simulink library "Libreria"  (R2019a)
settings: Solver=VariableStepAuto  StartTime=0.0  StopTime=10.0  RelTol=1e-3
values from neighbouring files (symbols this model uses):
  T_muestreo = 1    [Inicializacion_datos_distrito_personalizado.m]    (also in Inicializacion_datos_invernadero_tradicional.m; Inicializacion_datos_microred.m; Inicializacion_datos_nanofiltracion.m; Inicializacion_datos_oficinas.m)
undefined symbols (not defined in the file or in its folder): beta1, dispatch_factor, efficiency, Max_in, Min_in, Tm
settings Model: Creator=Usuario  LastModifiedBy=Jero

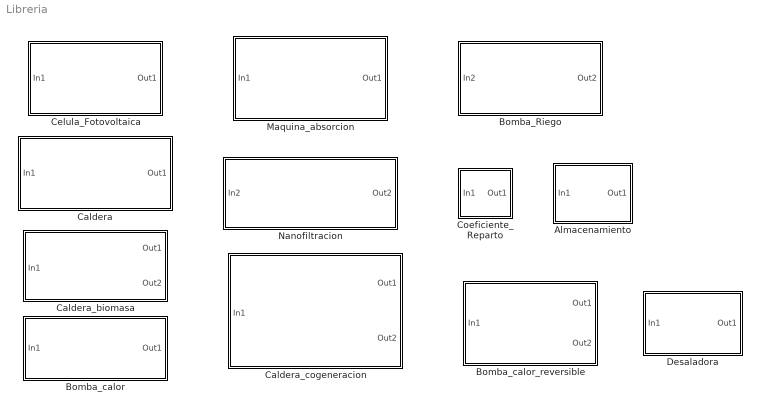
== system Libreria ==
  Almacenamiento : Subsystem  mask{Up2=1000, Low2=0, r_c=1, Up=1000, Low=0, r_d=1, Up1=1000, Low1=0, almacenamiento_inicial=0, cpa=1, almacenamiento_on=on}
      mask prompts: Up2 "Máximo"; Low2 "Mínimo"; r_c "rendimiento"; Up "Máximo"; Low "Mínimo"; r_d "rendimiento"; Up1 "Máximo"; Low1 "Mínimo"; almacenamiento_inicial "Condiciones iniciales"; cpa "Coeficiente de pérdidas"; almacenamiento_on "Almacenar energía"
      mask DialogControl DescGroupVar Prompt: Descripción
      mask DialogControl DescTextVar Prompt: Bloque de almacenamiento: se coloca en serie con la salida
      mask DialogControl ParameterGroupVar Prompt: Límites de los flujos de energía
      mask DialogControl Container6 Prompt: Carga
      mask DialogControl Container3 Prompt: Descarga
      mask DialogControl Container8 Prompt: Almacenamiento
      mask Display:
      | Ud = get_param(gcb,'UserData');
      | image(Ud.icono);
      | color('red');
  Bomba_Riego : Subsystem  mask{efficiency=1, dispatch_factor=beta1, T_muestreo=T_muestreo, Max_in=150, Max_out=150, n_salida=[0]}
      mask prompts: efficiency "Eficiencia"; dispatch_factor "Coeficiente de reparto"; T_muestreo "Tiempo de muestreo"; Max_in "Entrada"; Max_out "Salida"; n_salida "Salida asociada"
      mask TypeOptions efficiency: Ganancia_1_salida_max/efficiency
      mask TypeOptions dispatch_factor: Ganancia_1_salida_max/dispatch_factor
      mask TypeOptions T_muestreo: Ganancia_1_salida_max/T_muestreo
      mask TypeOptions Max_in: Ganancia_1_salida_max/Max_in
      mask DialogControl DescGroupVar Prompt: Descripción
      mask DialogControl DescTextVar Prompt: Su funcionamiento conlleva el uso de una demanda eléctrica en el energy hub. Representa el bombeamiento de agua para riego.
      mask DialogControl ParameterGroupVar Prompt: Parámetros
      mask DialogControl Container3 Prompt: Flujos máximos de energía
      mask DialogControl Container10 Prompt: Parámetros auxiliares
      mask Display:
      | ud=get_param(gcb,'UserData');
      | image(ud.icono);
      | color('green');
      | port_label('input',1,'IW');
      | port_label('output',1,'IW');
  Bomba_calor : Subsystem  mask{efficiency=[5.4], dispatch_factor=1, Tm=T_muestreo, Max_in=10, Max_out=54}
      mask prompts: efficiency "Eficiencia"; dispatch_factor "Coeficiente de reparto"; Tm "Tiempo de muestreo"; Max_in "Máximo"; Max_out "Máximo"
      mask TypeOptions efficiency: Ganancia_1_salida_max/efficiency
      mask TypeOptions dispatch_factor: Ganancia_1_salida_max/dispatch_factor
      mask TypeOptions Tm: Ganancia_1_salida_max/T_muestreo
      mask TypeOptions Max_in: Ganancia_1_salida_max/Max_in
      mask DialogControl DescGroupVar Prompt: Descripción
      mask DialogControl DescTextVar Prompt: Transforma energía eléctrica en calefacción.
      mask DialogControl ParameterGroupVar Prompt: Parámetros
      mask DialogControl Container3 Prompt: Límites de los flujos de energía
      mask DialogControl Container4 Prompt: Entrada
      mask DialogControl Container5 Prompt: Salida
      mask Display:
      | ud=get_param(gcb,'UserData');
      | image(ud.icono);
      | color('green');
      | port_label('input',1,'E');
      | color('red')
      | port_label('output',1,'H');
  Bomba_calor_reversible : Subsystem  mask{efficiency=efficiency, dispatch_factor=1, T_muestreo=T_muestreo, Max_in=Max_in, Min_in=Min_in, Max_out=[30 40], Salida_Binaria=[1 0]}
      mask prompts: efficiency "Eficiencia"; dispatch_factor "Coeficiente de reparto"; T_muestreo "Tiempo de muestreo"; Max_in "Máxima"; Min_in "Mínima"; Max_out "Máximo"; Salida_Binaria "Salidas Binarias:"
      mask TypeOptions efficiency: Ganancia_2_salidas/efficiency
      mask TypeOptions dispatch_factor: Ganancia_2_salidas/dispatch_factor
      mask TypeOptions T_muestreo: Ganancia_2_salidas/T_muestreo
      mask TypeOptions Max_in: Ganancia_2_salidas/Max_in
      mask TypeOptions Min_in: Ganancia_2_salidas/Min_in
      mask DialogControl DescGroupVar Prompt: Descripción
      mask DialogControl DescTextVar Prompt: Transforma energía eléctrica en refrigeración o calefacción. La transformación no se realiza simultáneamente.
      mask DialogControl ParameterGroupVar Prompt: Parámetros
      mask DialogControl Container3 Prompt: Límites de los flujos de energía
      mask DialogControl Container4 Prompt: Entrada
      mask DialogControl Container5 Prompt: Salida
      mask DialogControl Container6 Prompt: Parámetro auxiliar:
      mask DialogControl Control2 Prompt: Cambia durante la ejecución del optimizador. Sólo modifique este parámetro si va a realizar simulación sin optimizar previamente, en caso contrario no tendrá efecto la modificación.
      mask Display:
      | ud=get_param(gcb,'UserData');
      | image(ud.icono);
      | color('green');
      | port_label('input',1,'E');
      | color('blue');
      | port_label('output',1,'C');
      | color('red');
      | port_label('output',2,'H');
  Caldera : Subsystem  mask{efficiency=0, dispatch_factor=1, T_muestreo=T_muestreo, Min_in=0, Max_in=0, Max_out=1000}
      mask prompts: efficiency "Eficiencia"; dispatch_factor "Coeficiente de reparto"; T_muestreo "Tiempo de muestreo"; Min_in "Mínimo"; Max_in "Máximo"; Max_out "Máximo"
      mask TypeOptions efficiency: Ganancia_1_salida_max_min/efficiency
      mask TypeOptions dispatch_factor: Ganancia_1_salida_max_min/dispatch_factor
      mask TypeOptions T_muestreo: Ganancia_1_salida_max_min/T_muestreo
      mask TypeOptions Min_in: Ganancia_1_salida_max_min/Min_in
      mask TypeOptions Max_in: Ganancia_1_salida_max_min/Max_in
      mask DialogControl DescGroupVar Prompt: Descripción
      mask DialogControl DescTextVar Prompt: Transforma combustible en calefacción.
      mask DialogControl ParameterGroupVar Prompt: Parámetros
      mask DialogControl Container5 Prompt: Límites de los flujos de energía
      mask DialogControl Container6 Prompt: Entrada
      mask DialogControl Container7 Prompt: Salida
      mask Display:
      | Ud = get_param(gcb,'UserData');
      | image(Ud.icono);
      | color('black');
      | port_label('input',1,'F');
      | color('red')
      | port_label('output',1,'H');
  Caldera_biomasa : Subsystem  mask{efficiency=efficiency, dispatch_factor=dispatch_factor, T_muestreo=Tm, Max_in=Max_in, Min_in=Min_in, Max_out=0}
      mask prompts: efficiency "Eficiencia"; dispatch_factor "Coeficiente de reparto"; T_muestreo "Tiempo de muestreo"; Max_in "Entrada máxima"; Min_in "Entrada mínima"; Max_out "Máxima"
      mask TypeOptions efficiency: Ganancia_2_salidas/efficiency
      mask TypeOptions dispatch_factor: Ganancia_2_salidas/dispatch_factor
      mask TypeOptions T_muestreo: Ganancia_2_salidas/T_muestreo
      mask TypeOptions Max_in: Ganancia_2_salidas/Max_in
      mask TypeOptions Min_in: Ganancia_2_salidas/Min_in
      mask DialogControl DescGroupVar Prompt: Descripción
      mask DialogControl DescTextVar Prompt: Transforma el combustible en calefacción y captura el dióxido de carbono generado
      mask DialogControl ParameterGroupVar Prompt: Parámetros
      mask DialogControl Container7 Prompt: Flujos de energía
      mask DialogControl Container8 Prompt: Entrada
      mask DialogControl Container9 Prompt: Salida
      mask Display:
      | Ud = get_param(gcb,'UserData');
      | image(Ud.icono);
      | color('black');
      | port_label('input',1,'F');
      | color('red');
      | port_label('output',1,'H');
      | color('cyan');
      | port_label('output',2,'CO2');
  Caldera_cogeneracion : Subsystem  mask{efficiency=[10 10], dispatch_factor=1, Tm=T_muestreo, Max_in=1, Min_in=0, Max_out=[10 10]}
      mask prompts: efficiency "Eficiencia"; dispatch_factor "Coeficiente de reparto"; Tm "Tiempo de muestreo"; Max_in "Máxima"; Min_in "Mínima"; Max_out "Máxima"
      mask TypeOptions efficiency: Ganancia_2_salidas/efficiency
      mask TypeOptions dispatch_factor: Ganancia_2_salidas/dispatch_factor
      mask TypeOptions Tm: Ganancia_2_salidas/T_muestreo
      mask TypeOptions Max_in: Ganancia_2_salidas/Max_in
      mask TypeOptions Min_in: Ganancia_2_salidas/Min_in
      mask DialogControl DescGroupVar Prompt: Descripción
      mask DialogControl DescTextVar Prompt: Transforma combustible en energía eléctrica y calefacción simultáneamente.
      mask DialogControl ParameterGroupVar Prompt: Parámetros
      mask DialogControl Container3 Prompt: Flujos de energía
      mask DialogControl Container4 Prompt: Entrada
      mask DialogControl Container5 Prompt: Salida
      mask Display:
      | Ud = get_param(gcb,'UserData');
      | image(Ud.icono);
      | color('black');
      | port_label('input',1,'F');
      | color('green');
      | port_label('output',1,'E');
      | color('red');
      | port_label('output',2,'H');
  Celula_Fotovoltaica : Subsystem  mask{efficiency=[0.211], dispatch_factor=1, T_muestreo=T_muestreo, Max_in=1200, Max_out=2000}
      mask prompts: efficiency "Eficiencia"; dispatch_factor "Coeficiente de reparto"; T_muestreo "Tiempo de muestreo"; Max_in "Entrada"; Max_out "Salida"
      mask TypeOptions efficiency: Ganancia_1_salida_max/efficiency
      mask TypeOptions dispatch_factor: Ganancia_1_salida_max/dispatch_factor
      mask TypeOptions T_muestreo: Ganancia_1_salida_max/T_muestreo
      mask TypeOptions Max_in: Ganancia_1_salida_max/Max_in
      mask DialogControl DescGroupVar Prompt: Descripción
      mask DialogControl DescTextVar Prompt: En eficiencia se introduce el parámetro de eficiencia de cada panel y los flujos máximos son relativos a un panel.
      mask DialogControl ParameterGroupVar Prompt: Parámetros
      mask DialogControl Container3 Prompt: Flujos máximos
      mask Display:
      | Ud = get_param(gcb,'UserData');
      | image(Ud.icono);
      | color('yellow');
      | port_label('input',1,'R');
      | color('green');
      | port_label('output',1,'E');
  Coeficiente_Reparto : Subsystem  mask{dispatch_factor=1, Tm=T_muestreo, Max_out=inf, Max_in=inf, efficiency=1}
      mask prompts: dispatch_factor "Coeficiente de reparto"; Tm "Tiempo de muestreo"
      mask TypeOptions dispatch_factor: Funcion_coef_reparto/dispatch_factor
      mask TypeOptions Tm: Funcion_coef_reparto/Tm
      mask DialogControl DescGroupVar Prompt: Descripción
      mask DialogControl DescTextVar Prompt: Bloque Coeficiente de Reparto. Admite alfa o beta seguidos de un número: alfa1, alfa2...
      mask DialogControl ParameterGroupVar Prompt: Parámetros
      mask Display: disp('CR')
  Desaladora : Subsystem  mask{efficiency=1, dispatch_factor=beta1, T_muestreo=T_muestreo, Max_in=150, Max_out=150, n_salida=[0]}
      mask prompts: efficiency "Eficiencia"; dispatch_factor "Coeficiente de reparto"; T_muestreo "Tiempo de muestreo"; Max_in "Entrada"; Max_out "Salida"; n_salida "Salida asociada"
      mask TypeOptions efficiency: Ganancia_1_salida_max/efficiency
      mask TypeOptions dispatch_factor: Ganancia_1_salida_max/dispatch_factor
      mask TypeOptions T_muestreo: Ganancia_1_salida_max/T_muestreo
      mask TypeOptions Max_in: Ganancia_1_salida_max/Max_in
      mask DialogControl DescGroupVar Prompt: Descripción
      mask DialogControl DescTextVar Prompt: Su funcionamiento conlleva el uso de una demanda eléctrica en el energy hub. Representa el bombeamiento de agua para riego.
      mask DialogControl ParameterGroupVar Prompt: Parámetros
      mask DialogControl Container3 Prompt: Flujos máximos de energía
      mask DialogControl Container10 Prompt: Parámetros auxiliares
      mask Display:
      | ud=get_param(gcb,'UserData');
      | image(ud.icono);
      | color('green');
      | port_label('input',1,'SW');
      | color('cyan');
      | port_label('output',1,'IW');
  Maquina_absorcion : Subsystem  mask{efficiency=efficiency, dispatch_factor=1, Tm=T_muestreo, Min_in=Min_in, Max_in=Max_in, Max_out=70}
      mask prompts: efficiency "Eficiencia"; dispatch_factor "Coeficiente de reparto"; Tm "Tiempo de muestreo"; Min_in "Mínimo"; Max_in "Máximo"; Max_out "Máximo"
      mask TypeOptions efficiency: Ganancia_1_salida_max_min/efficiency
      mask TypeOptions dispatch_factor: Ganancia_1_salida_max_min/dispatch_factor
      mask TypeOptions Tm: Ganancia_1_salida_max_min/T_muestreo
      mask TypeOptions Min_in: Ganancia_1_salida_max_min/Min_in
      mask TypeOptions Max_in: Ganancia_1_salida_max_min/Max_in
      mask DialogControl DescGroupVar Prompt: Descripción
      mask DialogControl DescTextVar Prompt: Transforma calefacción en refrigeración mediante absorción
      mask DialogControl ParameterGroupVar Prompt: Parámetros
      mask DialogControl Container3 Prompt: Límites de los flujos de energía
      mask DialogControl Container4 Prompt: Entrada
      mask DialogControl Container5 Prompt: Salida
      mask Display:
      | ud=get_param(gcb,'UserData');
      | image(ud.icono);
      | color('blue');
      | port_label('output',1,'C');
      | color('red');
      | port_label('input',1,'H');
  Nanofiltracion : Subsystem  mask{efficiency=efficiency, dispatch_factor=beta1, T_muestreo=T_muestreo, Max_in=Max_in, Max_out=60, n_salida=0}
      mask prompts: efficiency "Eficiencia"; dispatch_factor "Coeficiente de reparto"; T_muestreo "Tiempo de muestreo"; Max_in "Entrada"; Max_out "Salida"; n_salida "Salida asociada"
      mask TypeOptions efficiency: Ganancia_1_salida_max/efficiency
      mask TypeOptions dispatch_factor: Ganancia_1_salida_max/dispatch_factor
      mask TypeOptions T_muestreo: Ganancia_1_salida_max/T_muestreo
      mask TypeOptions Max_in: Ganancia_1_salida_max/Max_in
      mask DialogControl DescGroupVar Prompt: Descripción
      mask DialogControl DescTextVar Prompt: Módulo de nanofiltración. Purifica el agua residual, potabilizándola. Debe de tener una salida asociada
      mask DialogControl ParameterGroupVar Prompt: Parámetros
      mask DialogControl Container3 Prompt: Flujos máximos de energía
      mask DialogControl Container4 Prompt: Parámetros auxiliares
      mask Display:
      | Ud = get_param(gcb,'UserData');
      | image(Ud.icono);
      | color('red');
      | port_label('input',1,'WW');
      | color('green')
      | port_label('output',1,'IW');

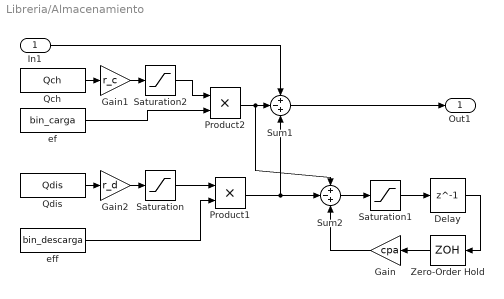
== system Libreria/Almacenamiento ==
  In1 : Inport
  Delay : Delay  DelayLength=1  InitialCondition=0
  Gain : Gain  Gain=cpa
  Gain1 : Gain  Gain=r_c
  Gain2 : Gain  Gain=r_d
  Product1 : Product
  Product2 : Product
  Qch : FromWorkspace  VariableName=Qch
  Qdis : FromWorkspace  VariableName=Qdis
  Saturation : Saturate  UpperLimit=Up  LowerLimit=Low
  Saturation1 : Saturate  UpperLimit=Up1  LowerLimit=Low1
  Saturation2 : Saturate  UpperLimit=Up2  LowerLimit=Low2
  Sum1 : Sum  Inputs=+-+
  Sum2 : Sum  Inputs=+-+
  Zero-Order Hold : ZeroOrderHold  SampleTime=-1
  ef : FromWorkspace  VariableName=bin_carga
  eff : FromWorkspace  VariableName=bin_descarga
  Out1 : Outport
  wires:
  Qdis/1 -> Gain2/1
  ef/1 -> Product2/2
  eff/1 -> Product1/2
  Saturation1/1 -> Delay/1
  In1/1 -> Sum1/1
  Sum1/1 -> Out1/1
  Sum2/1 -> Saturation1/1
  Delay/1 -> Zero-Order Hold/1
  Zero-Order Hold/1 -> Gain/1
  Gain/1 -> Sum2/3
  Qch/1 -> Gain1/1
  Gain1/1 -> Saturation2/1
  Gain2/1 -> Saturation/1
  Saturation/1 -> Product1/1
  Product1/1 -> Sum2/2, Sum1/3
  Saturation2/1 -> Product2/1
  Product2/1 -> Sum2/1, Sum1/2

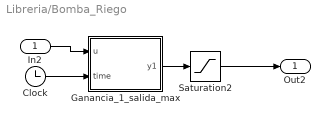
== system Libreria/Bomba_Riego ==
  In2 : Inport
  Clock : Clock
  Ganancia_1_salida_max : MATLAB Function  TreatAsAtomicUnit=on  mask{Max_in=Max_in, efficiency=efficiency, T_muestreo=T_muestreo, dispatch_factor=dispatch_factor}
      mask prompts: Max_in "Máximo"; efficiency "Eficiencia"; T_muestreo "Tiempo de muestreo"; dispatch_factor "Coeficiente de reparto"
  Saturation2 : Saturate  UpperLimit=Max_out  LowerLimit=-inf
  Out2 : Outport
  wires:
  Clock/1 -> Ganancia_1_salida_max/2(time)
  Saturation2/1 -> Out2/1
  In2/1 -> Ganancia_1_salida_max/1(u)
  Ganancia_1_salida_max/1(y1) -> Saturation2/1

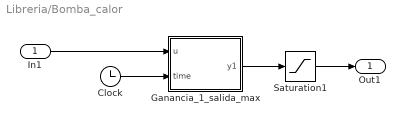
== system Libreria/Bomba_calor ==
  In1 : Inport
  Clock : Clock
  Ganancia_1_salida_max : MATLAB Function  TreatAsAtomicUnit=on  mask{Max_in=Max_in, efficiency=efficiency, T_muestreo=Tm, dispatch_factor=dispatch_factor}
      mask prompts: Max_in "Máximo"; efficiency "Eficiencia"; T_muestreo "Tiempo de muestreo"; dispatch_factor "Coeficiente de reparto"
  Saturation1 : Saturate  UpperLimit=Max_out(1)  LowerLimit=-inf
  Out1 : Outport
  wires:
  Saturation1/1 -> Out1/1
  Clock/1 -> Ganancia_1_salida_max/2(time)
  In1/1 -> Ganancia_1_salida_max/1(u)
  Ganancia_1_salida_max/1(y1) -> Saturation1/1

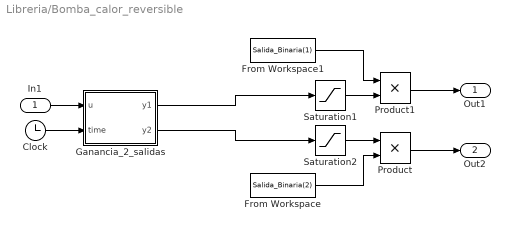
== system Libreria/Bomba_calor_reversible ==
  In1 : Inport
  Clock : Clock
  From Workspace : FromWorkspace  VariableName=Salida_Binaria(2)  SampleTime=0
  From Workspace1 : FromWorkspace  VariableName=Salida_Binaria(1)  SampleTime=0
  Ganancia_2_salidas : MATLAB Function  TreatAsAtomicUnit=on  mask{efficiency=efficiency, T_muestreo=T_muestreo, Max_in=Max_in, Min_in=Min_in, dispatch_factor=dispatch_factor}
      mask prompts: efficiency "Eficiencia"; T_muestreo "Tiempo de muestreo"; Max_in "Entrada máxima"; Min_in "Entrada mínima"; dispatch_factor "Coeficiente de reparto"
  Product : Product
  Product1 : Product
  Saturation1 : Saturate  UpperLimit=Max_out(1)  LowerLimit=-inf
  Saturation2 : Saturate  UpperLimit=Max_out(2)  LowerLimit=-inf
  Out1 : Outport
  Out2 : Outport  Port=2
  wires:
  In1/1 -> Ganancia_2_salidas/1(u)
  Clock/1 -> Ganancia_2_salidas/2(time)
  Ganancia_2_salidas/1(y1) -> Saturation1/1
  Ganancia_2_salidas/2(y2) -> Saturation2/1
  Product/1 -> Out2/1
  Saturation2/1 -> Product/1
  Saturation1/1 -> Product1/2
  Product1/1 -> Out1/1
  From Workspace/1 -> Product/2
  From Workspace1/1 -> Product1/1

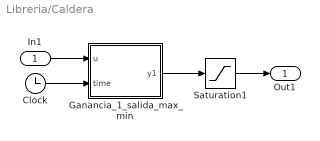
== system Libreria/Caldera ==
  In1 : Inport
  Clock : Clock
  Ganancia_1_salida_max_min : MATLAB Function  TreatAsAtomicUnit=on  mask{efficiency=efficiency, dispatch_factor=dispatch_factor, T_muestreo=T_muestreo, Min_in=Min_in, Max_in=Max_in}
      mask prompts: efficiency "Eficiencia"; dispatch_factor "Coeficiente de reparto"; T_muestreo "Tiempo de muestreo"; Min_in "Minimo de entrada"; Max_in "Minimo de salida"
  Saturation1 : Saturate  UpperLimit=Max_out  LowerLimit=-inf
  Out1 : Outport
  wires:
  Saturation1/1 -> Out1/1
  Ganancia_1_salida_max_min/1(y1) -> Saturation1/1
  Clock/1 -> Ganancia_1_salida_max_min/2(time)
  In1/1 -> Ganancia_1_salida_max_min/1(u)

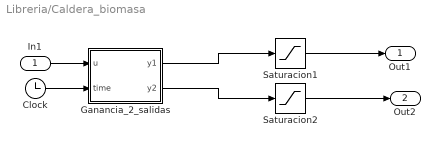
== system Libreria/Caldera_biomasa ==
  In1 : Inport
  Clock : Clock
  Ganancia_2_salidas : MATLAB Function  TreatAsAtomicUnit=on  mask{efficiency=efficiency, T_muestreo=T_muestreo, Max_in=Max_in, Min_in=Min_in, dispatch_factor=dispatch_factor}
      mask prompts: efficiency "Eficiencia"; T_muestreo "Tiempo de muestreo"; Max_in "Entrada máxima"; Min_in "Entrada mínima"; dispatch_factor "Coeficiente de reparto"
  Saturacion1 : Saturate  UpperLimit=Max_out(1)  LowerLimit=-inf
  Saturacion2 : Saturate  UpperLimit=Max_out(2)  LowerLimit=-inf
  Out1 : Outport
  Out2 : Outport  Port=2
  wires:
  Ganancia_2_salidas/2(y2) -> Saturacion2/1
  Ganancia_2_salidas/1(y1) -> Saturacion1/1
  Clock/1 -> Ganancia_2_salidas/2(time)
  In1/1 -> Ganancia_2_salidas/1(u)
  Saturacion2/1 -> Out2/1
  Saturacion1/1 -> Out1/1

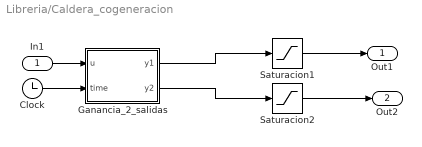
== system Libreria/Caldera_cogeneracion ==
  In1 : Inport
  Clock : Clock
  Ganancia_2_salidas : MATLAB Function  TreatAsAtomicUnit=on  mask{efficiency=efficiency, T_muestreo=Tm, Max_in=Max_in, Min_in=Min_in, dispatch_factor=dispatch_factor}
      mask prompts: efficiency "Eficiencia"; T_muestreo "Tiempo de muestreo"; Max_in "Entrada máxima"; Min_in "Entrada mínima"; dispatch_factor "Coeficiente de reparto"
  Saturacion1 : Saturate  UpperLimit=Max_out(1)  LowerLimit=-inf
  Saturacion2 : Saturate  UpperLimit=Max_out(2)  LowerLimit=-inf
  Out1 : Outport
  Out2 : Outport  Port=2
  wires:
  Saturacion1/1 -> Out1/1
  Saturacion2/1 -> Out2/1
  In1/1 -> Ganancia_2_salidas/1(u)
  Clock/1 -> Ganancia_2_salidas/2(time)
  Ganancia_2_salidas/1(y1) -> Saturacion1/1
  Ganancia_2_salidas/2(y2) -> Saturacion2/1

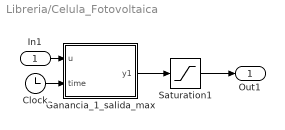
== system Libreria/Celula_Fotovoltaica ==
  In1 : Inport
  Clock : Clock
  Ganancia_1_salida_max : MATLAB Function  TreatAsAtomicUnit=on  mask{Max_in=Max_in, efficiency=efficiency, T_muestreo=T_muestreo, dispatch_factor=dispatch_factor}
      mask prompts: Max_in "Máximo"; efficiency "Eficiencia"; T_muestreo "Tiempo de muestreo"; dispatch_factor "Coeficiente de reparto"
  Saturation1 : Saturate  UpperLimit=Max_out  LowerLimit=-inf
  Out1 : Outport
  wires:
  Saturation1/1 -> Out1/1
  Ganancia_1_salida_max/1(y1) -> Saturation1/1
  In1/1 -> Ganancia_1_salida_max/1(u)
  Clock/1 -> Ganancia_1_salida_max/2(time)

== system Libreria/Coeficiente_Reparto ==
  In1 : Inport
  Clock : Clock
  Funcion_coef_reparto : MATLAB Function  TreatAsAtomicUnit=on  mask{dispatch_factor=dispatch_factor, Tm=Tm}
      mask prompts: dispatch_factor "Coeficiente de reparto"; Tm "Tiempo de muestreo"
  Out1 : Outport
  wires:
  In1/1 -> Funcion_coef_reparto/1(u)
  Clock/1 -> Funcion_coef_reparto/2(time)
  Funcion_coef_reparto/1(y) -> Out1/1

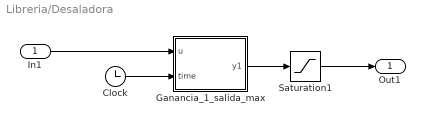
== system Libreria/Desaladora ==
  In1 : Inport
  Clock : Clock
  Ganancia_1_salida_max : MATLAB Function  TreatAsAtomicUnit=on  mask{Max_in=Max_in, efficiency=efficiency, T_muestreo=T_muestreo, dispatch_factor=dispatch_factor}
      mask prompts: Max_in "Máximo"; efficiency "Eficiencia"; T_muestreo "Tiempo de muestreo"; dispatch_factor "Coeficiente de reparto"
  Saturation1 : Saturate  UpperLimit=Max_out(1)  LowerLimit=-inf
  Out1 : Outport
  wires:
  In1/1 -> Ganancia_1_salida_max/1(u)
  Clock/1 -> Ganancia_1_salida_max/2(time)
  Ganancia_1_salida_max/1(y1) -> Saturation1/1
  Saturation1/1 -> Out1/1

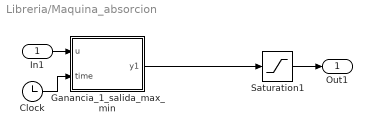
== system Libreria/Maquina_absorcion ==
  In1 : Inport
  Clock : Clock
  Ganancia_1_salida_max_min : MATLAB Function  TreatAsAtomicUnit=on  mask{efficiency=efficiency, dispatch_factor=dispatch_factor, T_muestreo=Tm, Min_in=Min_in, Max_in=Max_in}
      mask prompts: efficiency "Eficiencia"; dispatch_factor "Coeficiente de reparto"; T_muestreo "Tiempo de muestreo"; Min_in "Minimo de entrada"; Max_in "Minimo de salida"
  Saturation1 : Saturate  UpperLimit=Max_out  LowerLimit=-inf
  Out1 : Outport
  wires:
  In1/1 -> Ganancia_1_salida_max_min/1(u)
  Clock/1 -> Ganancia_1_salida_max_min/2(time)
  Ganancia_1_salida_max_min/1(y1) -> Saturation1/1
  Saturation1/1 -> Out1/1

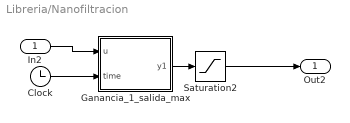
== system Libreria/Nanofiltracion ==
  In2 : Inport
  Clock : Clock
  Ganancia_1_salida_max : MATLAB Function  TreatAsAtomicUnit=on  mask{Max_in=Max_in, efficiency=efficiency, T_muestreo=T_muestreo, dispatch_factor=dispatch_factor}
      mask prompts: Max_in "Máximo"; efficiency "Eficiencia"; T_muestreo "Tiempo de muestreo"; dispatch_factor "Coeficiente de reparto"
  Saturation2 : Saturate  UpperLimit=Max_out  LowerLimit=-inf
  Out2 : Outport
  wires:
  Ganancia_1_salida_max/1(y1) -> Saturation2/1
  Saturation2/1 -> Out2/1
  In2/1 -> Ganancia_1_salida_max/1(u)
  Clock/1 -> Ganancia_1_salida_max/2(time)

== matlab function Libreria/Caldera/Ganancia_1_salida_max_min ==
  data: u input; y1 output; time input; Min_in parameter; Max_in parameter; efficiency parameter; T_muestreo parameter; dispatch_factor parameter
function y1  = fcn(u,time, Min_in, Max_in, efficiency, T_muestreo, dispatch_factor)
%efficiency: eficiencia
%Max_in: límite de entrada superior
%Min_in: límite de entrada inferior
%T_muestreo: tiempo de muestreo
%dispatch_factor: coeficiente de reparto
%time: tiempo de simulación
%u: entrada
%y1:salida
g=efficiency;
if(size(dispatch_factor,2)>1||size(g,1)>1)
    aux=floor(time/T_muestreo)+1;
    if(size(g,1)==1)
        u=min_max(u,dispatch_factor(aux),Max_in,Min_in)
        y1=u*dispatch_factor(aux)*g;
    end
    if(size(dispatch_factor,2)==1)
        u=min_max(u,dispatch_factor,Max_in,Min_in)
        y1=u*dispatch_factor*g(aux);
    end
else
    u=min_max(u,dispatch_factor,Max_in,Min_in)
    y1=u*dispatch_factor*g;
end
end

%obtengo los límites de entrada al dispositivo
function u=min_max(a,dispatch_factor,Max_in,Min_in)
if(a*dispatch_factor>Max_in)
    u=Max_in;
else
    u=a;
end
if(a*dispatch_factor<Min_in)
    u=Min_in;
else
    u=a;
end
end

== matlab function Libreria/Caldera_cogeneracion/Ganancia_2_salidas ==
  data: u input; y1 output; time input; y2 output; Min_in parameter; Max_in parameter; efficiency parameter; T_muestreo parameter; dispatch_factor parameter
function [y1,y2] = fcn(u,time, Min_in, Max_in, efficiency, T_muestreo, dispatch_factor)

%efficiency: eficiencia
%Max_in: límite de entrada superior
%Min_in: límite de entrada inferior
%T_muestreo: tiempo de muestreo
%dispatch_factor: coeficiente de reparto
%time: tiempo de simulación
%u: entrada
%y1: salida 1
%y2: salida 2

g=efficiency;
if(size(dispatch_factor,2)>1||size(g,1)>1)
    aux=floor(time/T_muestreo)+1;
    if(size(g,1)==1)
        u = max_min_u(u,dispatch_factor(aux),Min_in, Max_in);
        y1=u*dispatch_factor(aux)*g(1,1);
        y2=u*dispatch_factor(aux)*g(1,2);
    end
    if(size(dispatch_factor,2)==1)
        u = max_min_u(u,dispatch_factor, Min_in, Max_in);
        y1=u*dispatch_factor*g(aux,1);
        y2=u*dispatch_factor*g(aux,2);
    end
else
    u = max_min_u(u,dispatch_factor ,Min_in, Max_in);
    y1=u*dispatch_factor*g(1,1);
    y2=u*dispatch_factor*g(1,2);
end

end

% obtengo los límites de entrada de energía del dispositivo
function u = max_min_u(a,dispatch_factor, Min_in, Max_in)
if(a*dispatch_factor>Max_in)
    u=Max_in;
else
    u=a;
end
if(a*dispatch_factor<Min_in)
    u=Min_in;
else
    u=a;
end
end

== matlab function Libreria/Bomba_calor/Ganancia_1_salida_max ==
  data: u input; y1 output; time input; dispatch_factor parameter; T_muestreo parameter; efficiency parameter; Max_in parameter
function y1  = fcn(u,time, dispatch_factor, T_muestreo, efficiency, Max_in)
g=efficiency;

if(size(dispatch_factor,2)>1||size(g,1)>1)
    aux=floor(time/T_muestreo)+1;
    if(size(g,1)==1)
        u = max_min_u(u,dispatch_factor(aux), Max_in);
        y1=u*dispatch_factor(aux)*g;
    end
    if(size(dispatch_factor,2)==1)
        u = max_min_u(u,dispatch_factor,Max_in);
        y1=u*dispatch_factor*g(aux);
    end
else
    u = max_min_u(u,dispatch_factor,Max_in);
    y1=u*dispatch_factor*g;
end
end

% obtengo los límites de entrada de energía del dispositivo
function u = max_min_u(a,dispatch_factor,Max_in)
if(a*dispatch_factor>Max_in)
    u=Max_in;
else
    u=a;
end
end

== matlab function Libreria/Coeficiente_Reparto/Funcion_coef_reparto ==
  data: u input; y output; time input; dispatch_factor parameter; Tm parameter
function y = fcn(u,time, dispatch_factor, Tm)
%y: salida del bloque
%u: entrada 1 del bloque
%time: entrada 2 del bloque, tiempo de simulación
%dispatch_factor: vector coeficiente de reparto
%Tm: tiempo de muestreo
%Si el coeficiente de reparto no es un número
if(size(dispatch_factor,2)>1)
        %se obtiene la posición del vector en función del instante de muestreo
    aux=floor(time/Tm)+1;
    y=u*dispatch_factor(aux);
else
    %no se usa tiempo de muestreo
    y=u*dispatch_factor;
end

end

== matlab function Libreria/Maquina_absorcion/Ganancia_1_salida_max_min ==
  data: u input; y1 output; time input; Min_in parameter; Max_in parameter; efficiency parameter; T_muestreo parameter; dispatch_factor parameter
function y1  = fcn(u,time, Min_in, Max_in, efficiency, T_muestreo, dispatch_factor)
g=efficiency;
if(size(dispatch_factor,2)>1||size(g,1)>1)
    aux=floor(time/T_muestreo)+1;
    if(size(g,1)==1)
        u=min_max(u,dispatch_factor(aux),Max_in,Min_in)
        y1=u*dispatch_factor(aux)*g;
    end
    if(size(dispatch_factor,2)==1)
        u=min_max(u,dispatch_factor,Max_in,Min_in)
        y1=u*dispatch_factor*g(aux);
    end
else
    u=min_max(u,dispatch_factor,Max_in,Min_in)
    y1=u*dispatch_factor*g;
end
end

%obtengo los límites de entrada al dispositivo
function u=min_max(a,dispatch_factor,Max_in,Min_in)
if(a*dispatch_factor>Max_in)
    u=Max_in;
else
    u=a;
end
if(a*dispatch_factor<Min_in)
    u=Min_in;
else
    u=a;
end
end

== matlab function Libreria/Bomba_calor_reversible/Ganancia_2_salidas ==
  data: u input; y1 output; time input; y2 output; Min_in parameter; Max_in parameter; efficiency parameter; T_muestreo parameter; dispatch_factor parameter
function [y1,y2] = fcn(u,time, Min_in, Max_in, efficiency, T_muestreo, dispatch_factor)
g=efficiency;
if(size(dispatch_factor,2)>1||size(g,1)>1)
    aux=floor(time/T_muestreo)+1;
    if(size(g,1)==1)
        u = max_min_u(u,dispatch_factor(aux),Min_in, Max_in);
        y1=u*dispatch_factor(aux)*g(1,1);
        y2=u*dispatch_factor(aux)*g(1,2);
    end
    if(size(dispatch_factor,2)==1)
        u = max_min_u(u,dispatch_factor, Min_in, Max_in);
        y1=u*dispatch_factor*g(aux,1);
        y2=u*dispatch_factor*g(aux,2);
    end
else
    u = max_min_u(u,dispatch_factor ,Min_in, Max_in);
    y1=u*dispatch_factor*g(1,1);
    y2=u*dispatch_factor*g(1,2);
end

end

% obtengo los límites de entrada de energía del dispositivo
function u = max_min_u(a,dispatch_factor, Min_in, Max_in)
if(a*dispatch_factor>Max_in)
    u=Max_in;
else
    u=a;
end
if(a*dispatch_factor<Min_in)
    u=Min_in;
else
    u=a;
end
end

== matlab function Libreria/Nanofiltracion/Ganancia_1_salida_max ==
  data: u input; y1 output; time input; dispatch_factor parameter; T_muestreo parameter; efficiency parameter; Max_in parameter
function y1  = fcn(u,time, dispatch_factor, T_muestreo, efficiency, Max_in)
g=efficiency;

if(size(dispatch_factor,2)>1||size(g,1)>1)
    aux=floor(time/T_muestreo)+1;
    if(size(g,1)==1)
        u = max_min_u(u,dispatch_factor(aux), Max_in);
        y1=u*dispatch_factor(aux)*g;
    end
    if(size(dispatch_factor,2)==1)
        u = max_min_u(u,dispatch_factor,Max_in);
        y1=u*dispatch_factor*g(aux);
    end
else
    u = max_min_u(u,dispatch_factor,Max_in);
    y1=u*dispatch_factor*g;
end
end

% obtengo los límites de entrada de energía del dispositivo
function u = max_min_u(a,dispatch_factor,Max_in)
if(a*dispatch_factor>Max_in)
    u=Max_in;
else
    u=a;
end
end

== matlab function Libreria/Bomba_Riego/Ganancia_1_salida_max ==
  data: u input; y1 output; time input; dispatch_factor parameter; T_muestreo parameter; efficiency parameter; Max_in parameter
function y1  = fcn(u,time, dispatch_factor, T_muestreo, efficiency, Max_in)
g=efficiency;

if(size(dispatch_factor,2)>1||size(g,1)>1)
    aux=floor(time/T_muestreo)+1;
    if(size(g,1)==1)
        u = max_min_u(u,dispatch_factor(aux), Max_in);
        y1=u*dispatch_factor(aux)*g;
    end
    if(size(dispatch_factor,2)==1)
        u = max_min_u(u,dispatch_factor,Max_in);
        y1=u*dispatch_factor*g(aux);
    end
else
    u = max_min_u(u,dispatch_factor,Max_in);
    y1=u*dispatch_factor*g;
end
end

% obtengo los límites de entrada de energía del dispositivo
function u = max_min_u(a,dispatch_factor,Max_in)
if(a*dispatch_factor>Max_in)
    u=Max_in;
else
    u=a;
end
end

== matlab function Libreria/Caldera_biomasa/Ganancia_2_salidas ==
  data: u input; y1 output; time input; y2 output; Min_in parameter; Max_in parameter; efficiency parameter; T_muestreo parameter; dispatch_factor parameter
function [y1,y2] = fcn(u,time, Min_in, Max_in, efficiency, T_muestreo, dispatch_factor)

%efficiency: eficiencia
%Max_in: límite de entrada superior
%Min_in: límite de entrada inferior
%T_muestreo: tiempo de muestreo
%dispatch_factor: coeficiente de reparto
%time: tiempo de simulación
%u: entrada
%y1: salida 1
%y2: salida 2

g=efficiency;
if(size(dispatch_factor,2)>1||size(g,1)>1)
    aux=floor(time/T_muestreo)+1;
    if(size(g,1)==1)
        u = max_min_u(u,dispatch_factor(aux),Min_in, Max_in);
        y1=u*dispatch_factor(aux)*g(1,1);
        y2=u*dispatch_factor(aux)*g(1,2);
    end
    if(size(dispatch_factor,2)==1)
        u = max_min_u(u,dispatch_factor, Min_in, Max_in);
        y1=u*dispatch_factor*g(aux,1);
        y2=u*dispatch_factor*g(aux,2);
    end
else
    u = max_min_u(u,dispatch_factor ,Min_in, Max_in);
    y1=u*dispatch_factor*g(1,1);
    y2=u*dispatch_factor*g(1,2);
end

end

% obtengo los límites de entrada de energía del dispositivo
function u = max_min_u(a,dispatch_factor, Min_in, Max_in)
if(a*dispatch_factor>Max_in)
    u=Max_in;
else
    u=a;
end
if(a*dispatch_factor<Min_in)
    u=Min_in;
else
    u=a;
end
end

== matlab function Libreria/Celula_Fotovoltaica/Ganancia_1_salida_max ==
  data: u input; y1 output; time input; dispatch_factor parameter; T_muestreo parameter; efficiency parameter; Max_in parameter
function y1  = fcn(u,time, dispatch_factor, T_muestreo, efficiency, Max_in)
%efficiency: eficiencia
%Max_in: límite de entrada superior
%T_muestreo: tiempo de muestreo
%dispatch_factor: coeficiente de reparto
%time: tiempo de simulación
%u: entrada
%y1:salida

g=efficiency;

if(size(dispatch_factor,2)>1||size(g,1)>1)
    aux=floor(time/T_muestreo)+1;
    if(size(g,1)==1)
        u = max_min_u(u,dispatch_factor(aux), Max_in);
        y1=u*dispatch_factor(aux)*g;
    end
    if(size(dispatch_factor,2)==1)
        u = max_min_u(u,dispatch_factor,Max_in);
        y1=u*dispatch_factor*g(aux);
    end
else
    u = max_min_u(u,dispatch_factor,Max_in);
    y1=u*dispatch_factor*g;
end
end

% obtengo los límites de entrada de energía del dispositivo
function u = max_min_u(a,dispatch_factor,Max_in)
if(a*dispatch_factor>Max_in)
    u=Max_in;
else
    u=a;
end
end

== matlab function Libreria/Desaladora/Ganancia_1_salida_max ==
  data: u input; y1 output; time input; dispatch_factor parameter; T_muestreo parameter; efficiency parameter; Max_in parameter
function y1  = fcn(u,time, dispatch_factor, T_muestreo, efficiency, Max_in)
g=efficiency;

if(size(dispatch_factor,2)>1||size(g,1)>1)
    aux=floor(time/T_muestreo)+1;
    if(size(g,1)==1)
        u = max_min_u(u,dispatch_factor(aux), Max_in);
        y1=u*dispatch_factor(aux)*g;
    end
    if(size(dispatch_factor,2)==1)
        u = max_min_u(u,dispatch_factor,Max_in);
        y1=u*dispatch_factor*g(aux);
    end
else
    u = max_min_u(u,dispatch_factor,Max_in);
    y1=u*dispatch_factor*g;
end
end

% obtengo los límites de entrada de energía del dispositivo
function u = max_min_u(a,dispatch_factor,Max_in)
if(a*dispatch_factor>Max_in)
    u=Max_in;
else
    u=a;
end
end
